simulink model "untitled"  (R2015b)
settings: Solver=VariableStepAuto  StartTime=0.0  StopTime=100.0  RelTol=1e-3
settings Model: Creator=dell  LastModifiedBy=dell

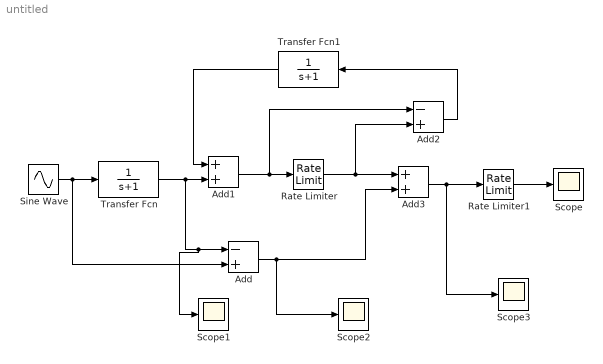
== system untitled ==
  Add : Sum  Inputs=-+
  Add1 : Sum
  Add2 : Sum  Inputs=-+
  Add3 : Sum
  Rate Limiter : RateLimiter  SampleTimeMode=inherited
  Rate Limiter1 : RateLimiter  SampleTimeMode=inherited
  Scope{,1..3} (4 alike) : Scope
  Sine Wave : Sin  SampleTime=0
  Transfer Fcn : TransferFcn  Denominator=[1 1]
  Transfer Fcn1 : TransferFcn  Denominator=[1 1]
  wires:
  Sine Wave/1 -> Add/2, Transfer Fcn/1
  Transfer Fcn/1 -> Scope1/1, Add/1, Add1/2
  Add1/1 -> Add2/1, Rate Limiter/1
  Rate Limiter/1 -> Add2/2, Add3/1
  Add/1 -> Scope2/1, Add3/2
  Add3/1 -> Scope3/1, Rate Limiter1/1
  Add2/1 -> Transfer Fcn1/1
  Transfer Fcn1/1 -> Add1/1
  Rate Limiter1/1 -> Scope/1
